simulink model "Ultrasonic"  (R2024a)
settings: Solver=FixedStepAuto  StartTime=0.0  StopTime=inf  FixedStep=0.0001  RelTol=1e-3
undefined symbols (not defined in the file or in its folder): DiscIntNeverNeededParam
libraries: dspsigops x3, bbblueBasicLib x2, spsFirstOrderFilterLib x1, simulink_extras x1, dspswit3 x1
settings Model: ExtModeTrigDuration=100  Creator=felih  LastModifiedBy=felih
settings SolverCC: PositivePriorityOrder=on  AutoInsertRateTranBlk=on
settings OptimizationCC: EnhancedBackFolding=on  PassReuseOutputArgsAs=Individual arguments  ZeroExternalMemoryAtStartup=off  ZeroInternalMemoryAtStartup=off  MaxStackSize=64  OptimizeBlockOrder=speed  DifferentSizesBufferReuse=on  OptimizationCustomize=off  EfficientTunableParamExpr=on
settings DebuggingCC: ParameterTunabilityLossMsg=error
settings HardwareCC: ProdBitPerPointer=32  ProdBitPerSizeT=32  ProdBitPerPtrDiffT=32  ProdLargestAtomicInteger=Long  ProdLargestAtomicFloat=Double  ProdWordSize=32  ProdHWDeviceType=ARM Compatible->ARM Cortex
settings SFSimCC: MATLABDynamicMemAlloc=off
settings RTWCC: Description=Embedded Coder  SystemTargetFile=ert.tlc  HardwareBoard=BeagleBone Blue  TLCOptions="-aInlineSetEventsForThisBaseRateFcn=TLC_FALSE -aSuppressMultiTaskScheduler=TLC_FALSE  -aRateBasedStepFcn=0"  TemplateMakefile=ert_default_tmf  Toolchain=GNU GCC BeagleBone Blue
settings CodeAppCC: ForceParamTrailComments=on  IgnoreCustomStorageClasses=off  OperatorAnnotations=on  SimulinkDataObjDesc=on  SFDataObjDesc=on  InsertBlockDesc=on
settings ERTTargetCC: SupportVariableSizeSignals=on

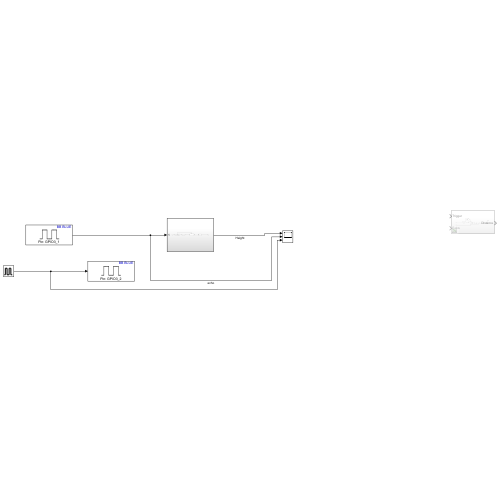
[thumbnail: Simulink's stored preview of the top-level diagram]
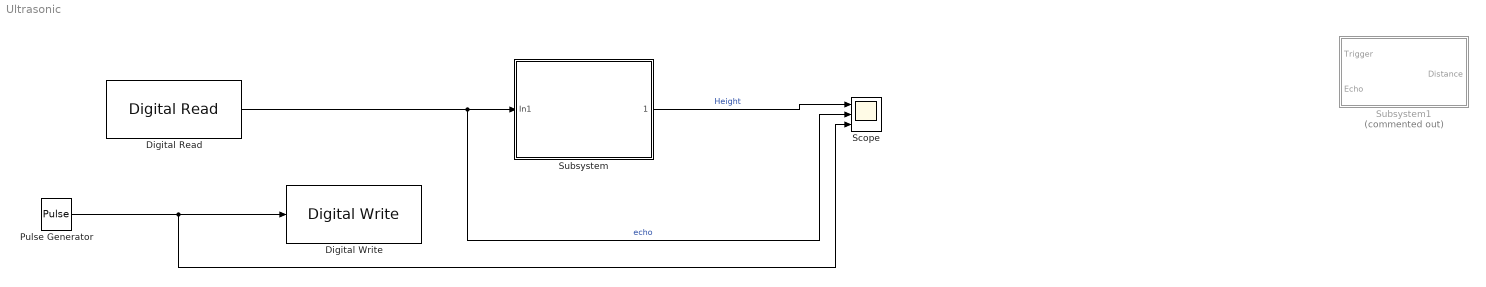
== system Ultrasonic ==
  Digital Read : bbblueBasicLib/Digital Read  Pin=49  Direction=input  GPIOSelect=GPIO3_1  SampleTime=0.0001
  Digital Write : bbblueBasicLib/Digital Write  GPIOSelect=GPIO3_2  Pin=49  Direction=output
  Pulse Generator : DiscretePulseGenerator  PulseType=Time based  Period=0.1  PulseWidth=10
  Scope : Scope  NumInputPorts=3
  Subsystem : Subsystem
  Subsystem1 : Subsystem  Commented=on
  wires:
  Subsystem/1(" ") -> Scope/1  "Height"
  Digital Read/1 -> Scope/2, Subsystem/1(In1)  "echo"
  Pulse Generator/1 -> Digital Write/1, Scope/3

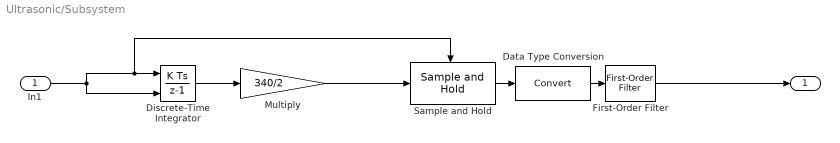
== system Ultrasonic/Subsystem ==
  In1 : Inport
  Data Type Conversion : DataTypeConversion  SaturateOnIntegerOverflow=off  RndMeth=Floor
  Discrete-Time Integrator : DiscreteIntegrator  ExternalReset=falling  SampleTime=-1  ICPrevOutput=DiscIntNeverNeededParam  ICPrevScaledInput=DiscIntNeverNeededParam
  First-Order Filter : spsFirstOrderFilterLib/First-Order Filter  FilterType=Lowpass  Tc=0.1  Ts=0.01  Initialize=off  Vac_Init=[0, 0, 60]  Vdc_Init=0  PlotResponse=off  FreqRange="[0,  200,  1]"
  Multiply : Gain  Gain=340/2
  Sample and Hold : dspsigops/Sample and Hold  trig=Falling edge  initCond=0  latchinput=on
  " " : Outport
  wires:
  Discrete-Time Integrator/1 -> Multiply/1
  In1/1 -> Sample and Hold/Trigger, Discrete-Time Integrator/1, Discrete-Time Integrator/2
  Multiply/1 -> Sample and Hold/1
  Data Type Conversion/1 -> First-Order Filter/1
  First-Order Filter/1 -> " "/1
  Sample and Hold/1 -> Data Type Conversion/1

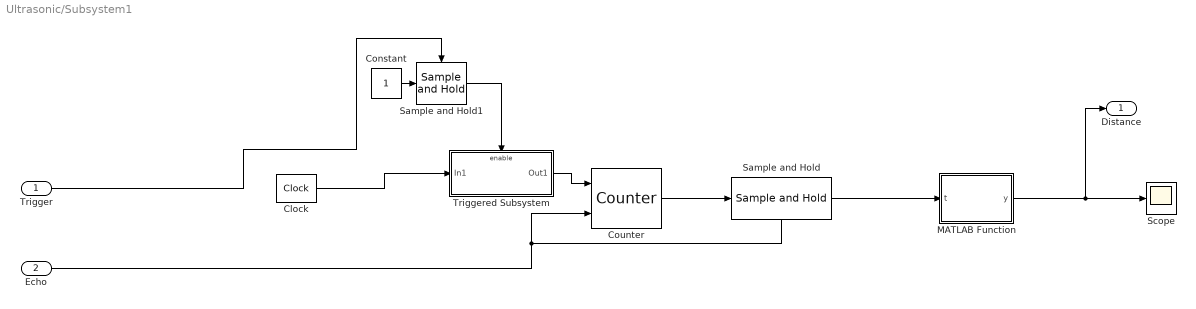
== system Ultrasonic/Subsystem1 ==
  Trigger : Inport
  Echo : Inport  Port=2
  Clock : simulink_extras/Flip Flops/Clock  period=0.001
  Constant : Constant
  Counter : dspswit3/Counter  Direction=Up  CountEvent=Rising edge  CounterSize=32 bits  MaxCount=255  InitialCount=0  Output=Count  HitValue=32  ResetInput=on  SamplesPerFrame=1  Ts=1  CntDtype=double  HitDtype=Logical
  MATLAB Function : MATLAB Function  TreatAsAtomicUnit=on
  Sample and Hold : dspsigops/Sample and Hold  trig=Rising edge  initCond=0  latchinput=on
  Sample and Hold1 : dspsigops/Sample and Hold  trig=Rising edge  initCond=0  latchinput=off
  Scope : Scope
  Triggered Subsystem : Subsystem  TreatAsAtomicUnit=on
  Distance : Outport
  wires:
  Sample and Hold/1 -> MATLAB Function/1(t)
  Sample and Hold1/1 -> Triggered Subsystem/Enable
  Triggered Subsystem/1(Out1) -> Counter/1
  Echo/1 -> Sample and Hold/Trigger, Counter/2
  Trigger/1 -> Sample and Hold1/Trigger
  Constant/1 -> Sample and Hold1/1
  Clock/1 -> Triggered Subsystem/1(In1)
  Counter/1 -> Sample and Hold/1
  MATLAB Function/1(y) -> Distance/1, Scope/1

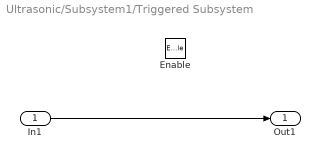
== system Ultrasonic/Subsystem1/Triggered Subsystem ==
  In1 : Inport
  Enable : EnablePort
  Out1 : Outport
  wires:
  In1/1 -> Out1/1

== matlab function Ultrasonic/Subsystem1/MATLAB Function ==
  data: t input; y output
function y = fcn(t)



y = ((t/1000)*340)/2;
